simulink model "mainModel_matlab2013a"  (R2016b)
settings: Solver=ode45  StartTime=0.0  StopTime=1000  RelTol=1e-3
settings Model: SimulationMode=rapid-accelerator  Creator=manoj  LastModifiedBy=manoj
settings DataIOCC: SaveFormat=StructureWithTime
settings OptimizationCC: LifeSpan=inf
settings DebuggingCC: SFExecutionAtInitializationDiag=none
settings HardwareCC: ProdBitPerSizeT=32  ProdBitPerPtrDiffT=32  ProdWordSize=32  ProdHWDeviceType=Specified

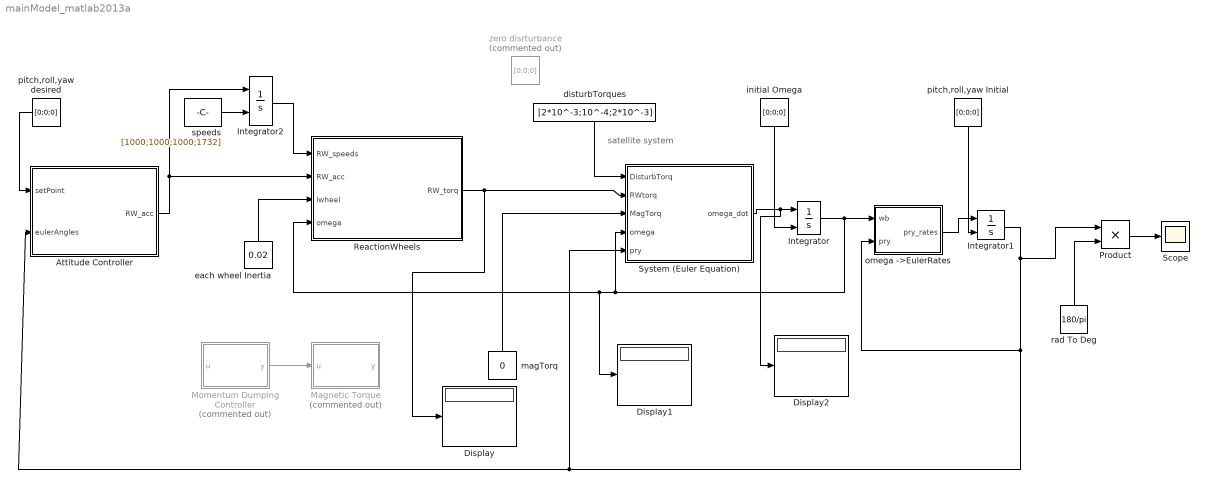
== system mainModel_matlab2013a ==
  note: satellite system
  "Attitude Controller " : MATLAB Function  TreatAsAtomicUnit=on
  Display : Display
  Display1 : Display
  Display2 : Display
  Integrator : Integrator  InitialConditionSource=external
  Integrator1 : Integrator  InitialConditionSource=external
  Integrator2 : Integrator  InitialConditionSource=external  LimitOutput=on  UpperSaturationLimit=2000  LowerSaturationLimit=100
  "Magnetic Torque " : MATLAB Function  Commented=on  TreatAsAtomicUnit=on
  Momentum Dumping Controller : MATLAB Function  Commented=on  TreatAsAtomicUnit=on
  Product : Product
  ReactionWheels : MATLAB Function  TreatAsAtomicUnit=on
  Scope : Scope
  "System (Euler Equation) " : MATLAB Function  TreatAsAtomicUnit=on
  disturbTorques : Constant  Value=[2*10^-3;10^-4;2*10^-3]
  each wheel Inertia : Constant  Value=0.02
  initial Omega : Constant  Value=[0;0;0]
  "magTorq " : Constant  Value=0
  omega ->EulerRates : MATLAB Function  TreatAsAtomicUnit=on
  pitch,roll,yaw Initial : Constant  Value=[0;0;0]
  pitch,roll,yaw desired : Constant  Value=[0;0;0]
  rad To Deg : Constant  Value=180/pi
  speeds : Constant  Value=[1000;1000;1000;1732]
  "zero disrturbance " : Constant  Commented=on  Value=[0;0;0]
  wires:
  "Attitude Controller "/1(RW_acc) -> Integrator2/1, ReactionWheels/2(RW_acc)
  Momentum Dumping Controller/1(y) -> "Magnetic Torque "/1(u)
  each wheel Inertia/1 -> ReactionWheels/3(Iwheel)
  Integrator2/1 -> ReactionWheels/1(RW_speeds)
  speeds/1 -> Integrator2/2
  pitch,roll,yaw desired/1 -> "Attitude Controller "/1(setPoint)
  Integrator/1 -> "System (Euler Equation) "/4(omega), Display1/1, ReactionWheels/4(omega), omega ->EulerRates/1(wb)
  Integrator1/1 -> Product/1, omega ->EulerRates/2(pry), "System (Euler Equation) "/5(pry), "Attitude Controller "/2(eulerAngles)
  ReactionWheels/1(RW_torq) -> Display/1, "System (Euler Equation) "/2(RWtorq)
  omega ->EulerRates/1(pry_rates) -> Integrator1/1
  "magTorq "/1 -> "System (Euler Equation) "/3(MagTorq)
  initial Omega/1 -> Integrator/2
  pitch,roll,yaw Initial/1 -> Integrator1/2
  Product/1 -> Scope/1
  rad To Deg/1 -> Product/2
  "System (Euler Equation) "/1(omega_dot) -> Display2/1, Integrator/1
  disturbTorques/1 -> "System (Euler Equation) "/1(DisturbTorq)

== matlab function mainModel_matlab2013a/Attitude Controller  ==
  data: setPoint input; eulerAngles input; RW_acc output
function RW_acc = fcn(setPoint,eulerAngles)
RW_acc=[0;0;0;0]; %no controller for now. This acceleration correspond
% to the rate of change in speed of each wheel. wheel speeds are always
% positive buy convention

end

== matlab function mainModel_matlab2013a/System (Euler Equation)  ==
  data: DisturbTorq input; RWtorq input; omega_dot output; MagTorq input; omega input; pry input
function omega_dot = fcn( DisturbTorq,RWtorq,MagTorq,omega,pry)
%[x,y,z] corresponds to yaw roll and pitch axis!!!
MOI=[1800 -50 -15;-50 1600 25;-15 25 1200];%momentOfInertia of Satellite(with everything)
%Mass=1600;%kg
p=pry(1);
r=pry(2);
y=pry(3);
Cx=[    1, 0, 0
        0, cos(y), sin(y)
        0, -sin(y), cos(y)    ];

Cy=[    cos(r), 0, -sin(r);
        0, 1, 0;
        sin(r), 0, cos(r) ];

Cz=[    cos(p), sin(p), 0;
        -sin(p), cos(p), 0;
        0, 0, 1    ];
Cbo=Cx*Cy*Cz; %orbit to body frame matrix adopting 3,2,1 convention on (x,y,z)
Wo=1.0741*10^-3;
temp1=(omega-Cbo*[0;0;Wo]);
omega_dot=(MOI)\(DisturbTorq+MagTorq-RWtorq-cross(temp1,MOI*temp1));

end

== matlab function mainModel_matlab2013a/Magnetic Torque  ==
  data: u input; y output
function y = fcn(u)

y = u;

== matlab function mainModel_matlab2013a/omega ->EulerRates ==
  data: wb input; pry_rates output; pry input
function pry_rates  = fcn(wb,pry)
%[x,y,z] 3-2-1 rotation, where x=yaw,y=roll,z=pitch axis
% pry-pitch,yaw,roll angles

% Cx=[    1, 0, 0
%         0, cos(yaw), sin(yaw)
%         0, -sin(yaw), cos(yaw)    ];
% 
% Cy=[    cos(roll), 0, -sin(roll);
%         0, 1, 0;
%         sin(roll), 0, cos(roll) ];
% 
% Cz=[    cos(pitch), sin(pitch), 0;
%         -sin(pitch), cos(pitch), 0;
%         0, 0, 1    ];NOT NEEDED HERE BUT CAN BE USED ELSEWHERE IF NEEDEd

%p=pry(1);
r=pry(2);
y=pry(3);
C_pryToOmega=   [   -sin(r),        0,      1
                    cos(r)*sin(y),  cos(y), 0
                    cos(r)*cos(y), -sin(y), 0];
pry_rates=(C_pryToOmega)\wb;

== matlab function mainModel_matlab2013a/ReactionWheels ==
  data: RW_speeds input; RW_acc input; RW_torq output; Iwheel input; omega input
function RW_torq = fcn(RW_speeds,RW_acc,Iwheel,omega)
%For Normal arrangement(not the tetrahedron one)
%RW_acc means acceleration of 4 individual wheel speeds

Torq_acceleration_part=Iwheel*[  RW_acc(1)-1/sqrt(3)*RW_acc(4);
                            RW_acc(2)-1/sqrt(3)*RW_acc(4);
                            RW_acc(3)-1/sqrt(3)*RW_acc(4)  ];
Torq_gyroscopic_part=Iwheel*[ RW_speeds(3)*omega(2)- RW_speeds(2)*omega(3);
                              RW_speeds(1)*omega(3)- RW_speeds(3)*omega(1);
                              RW_speeds(2)*omega(1)- RW_speeds(1)*omega(2)];
RW_torq=Torq_acceleration_part+Torq_gyroscopic_part;%gyroscopic part is actually undesired but still present                            
end

== matlab function mainModel_matlab2013a/Momentum Dumping Controller ==
  data: u input; y output
function y = fcn(u)

y = u;
